simulink model "TRGC_Lock_Unlock_Shifter"  (Simulink 7.8)
settings: Solver=ode45  StartTime=0.0  StopTime=10.0  RelTol=1e-3
undefined symbols (not defined in the file): CeTRGR_e_TransRangePark
libraries: ChryslerLib x2
settings Model: Creator=T6684MB  LastModifiedBy=T6684MB

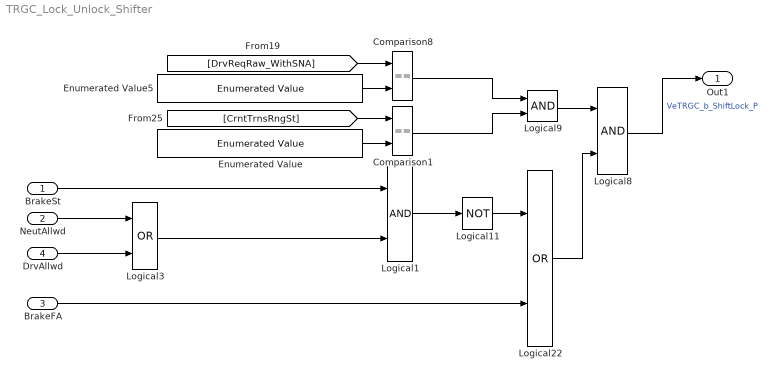
== system TRGC_Lock_Unlock_Shifter ==
  BrakeSt : Inport
  NeutAllwd : Inport  Port=2
  BrakeFA : Inport  Port=3
  DrvAllwd : Inport  Port=4
  Comparison1 : RelationalOperator  Operator===  OutDataTypeStr=boolean
  Comparison8 : RelationalOperator  Operator===  OutDataTypeStr=boolean
  Enumerated Value : ChryslerLib/Parameters & Constants/Enumerated Value  Value=CeTRGR_e_TransRangePark  OutMin=[]  OutMax=[]  OutDataTypeStr=TeTRGR_e_TransRangeState
  Enumerated Value5 : ChryslerLib/Parameters & Constants/Enumerated Value  Value=CeTRGR_e_TransRangePark  OutMin=[]  OutMax=[]  OutDataTypeStr=TeTRGR_e_TransRangeState
  Logical1 : Logic  OutDataTypeStr=boolean
  Logical11 : Logic  Operator=NOT  OutDataTypeStr=boolean
  Logical22 : Logic  Operator=OR  OutDataTypeStr=boolean
  Logical3 : Logic  Operator=OR  OutDataTypeStr=boolean
  Logical8 : Logic  OutDataTypeStr=boolean
  Logical9 : Logic  OutDataTypeStr=boolean
  Out1 : Outport
  wires:
  Logical3/1 -> Logical1/2
  DrvAllwd/1 -> Logical3/2
  NeutAllwd/1 -> Logical3/1
  BrakeSt/1 -> Logical1/1
  BrakeFA/1 -> Logical22/2
  Logical8/1 -> Out1/1  "VeTRGC_b_ShiftLock_P"
  Logical22/1 -> Logical8/2
  Logical11/1 -> Logical22/1
  Logical1/1 -> Logical11/1
  Logical9/1 -> Logical8/1
  [CrntTrnsRngSt] -> Comparison1/1
  Comparison1/1 -> Logical9/2
  Comparison8/1 -> Logical9/1
  [DrvReqRaw_WithSNA] -> Comparison8/1
  Enumerated Value5/1 -> Comparison8/2
  Enumerated Value/1 -> Comparison1/2
